simulink model "washingmachin"  (R2024b)
settings: Solver=VariableStepAuto  StartTime=0.0  StopTime=50  RelTol=1e-3
settings Model: Creator=sushm  LastModifiedBy=sushm

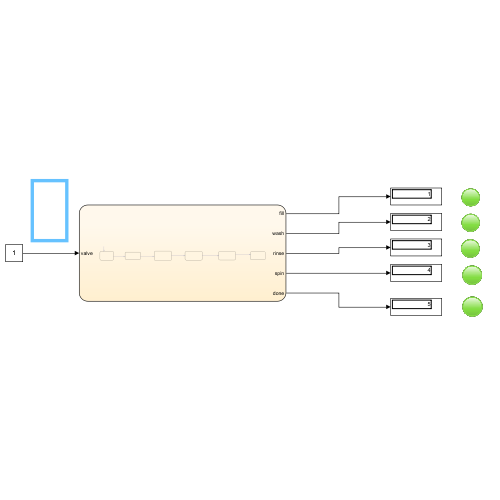
[thumbnail: Simulink's stored preview of the top-level diagram]
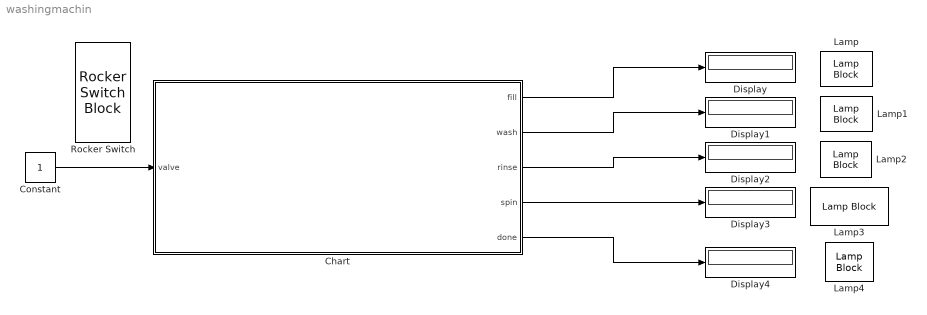
== system washingmachin ==
  Chart : Stateflow chart  TreatAsAtomicUnit=on
      settings: PortSchema="{\"entries\":[{\"content\":{\"sides\":[{\"content\":{\"connectorIds\":[\"In1\"]},\"type\":\"ConnectorPlacement.EquallySpacedRectSide\",\"uuid\":\"b717e67b-7bc3-4778-a1ab-25a0ceadf715\"},{\"content\":{\"connectorIds\":[\"Out2\",\"Out3\",\"Out5\",\"Out4\",\"Out1\"],\"side\":\"RIGHT\"},\"type\":\"ConnectorPlacement.EquallySpacedRectSide\",\"uuid\":\"15731e6c-0ddb-4397-bc3d-b35300a730c1\"},{\"content\":{\"side\":\"TOP\"},\"type\":\"ConnectorPlacement.EquallySpacedRectSide\",\"uuid\":\"788ecb44-8806-4dc9-b193-f08ea584cdf1\"}]},\"type\":\"ConnectorPlacement.EquallySpacedConnector\",\"uuid\":\"6bf343f3-e448-47f4-9ac8-0bf6f246dd38\"}],\"packageUris\":[\"http://schema.mathworks.com/mf0/Connector/R2020b\"],\"version\":\"1.0\"}"
  Constant : Constant
  Display{,1..4} (5 alike) : Display
  Lamp{,1..4} (5 alike) : LampBlock  LabelPosition=Hide
  Rocker Switch : RockerSwitchBlock
      settings: Values={{'Off', 'On'}, [0 1]}
  wires:
  Chart/2(fill) -> Display/1
  Chart/3(wash) -> Display1/1
  Constant/1 -> Chart/1(valve)
  Chart/5(rinse) -> Display2/1
  Chart/4(spin) -> Display3/1
  Chart/1(done) -> Display4/1

== stateflow chart washingmachin/Chart ==
  state wash
    entry: wash= 2
  state valve
  state rinse
    entry: rinse=3
  state spin
    entry: spin=4
  state done
    entry: done= 5
  state fill
    entry:fill=1
  (default) -> valve
  spin -> done : [after(10,sec)]
  wash -> rinse : [after(10,sec)]
  rinse -> spin : [after(10,sec)]
  valve -> fill : [valve==1]
  fill -> wash : [after(10,sec)]
  data: valve input; done output; fill output; wash output; spin output; rinse output
